simulink model "friction_compensation_test"  (R2022b)
settings: Solver=VariableStepAuto  StartTime=0.0  StopTime=10.0  RelTol=1e-3
values from neighbouring files (symbols this model uses):
  error_min = 0.04    [matlab.mat]
  pwm_k = 0.02    [matlab.mat]
  pwm_min = 0.27    [matlab.mat]
settings Model: Creator=sjohnson  LastModifiedBy=sjohnson

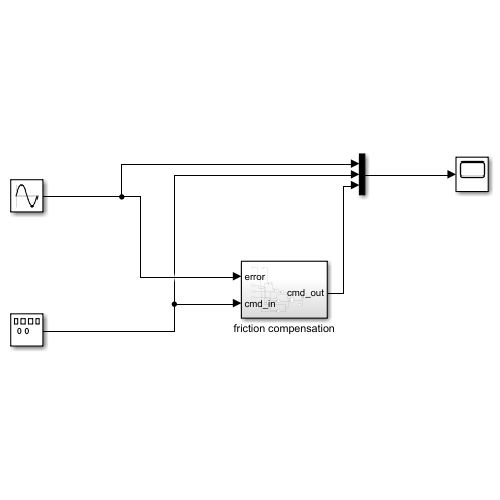
[thumbnail: Simulink's stored preview of the top-level diagram]
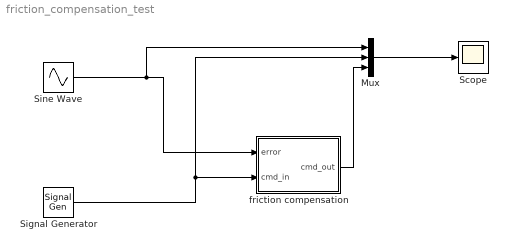
== system friction_compensation_test ==
  Mux : Mux  Inputs=3
  Scope : Scope
  Signal Generator : SignalGenerator  WaveForm=sawtooth  Units=rad/sec
  Sine Wave : Sin  SampleTime=0
  friction compensation : Subsystem
  wires:
  Sine Wave/1 -> Mux/1, friction compensation/1(error)
  Signal Generator/1 -> Mux/2, friction compensation/2(cmd_in)
  friction compensation/1(cmd_out) -> Mux/3
  Mux/1 -> Scope/1

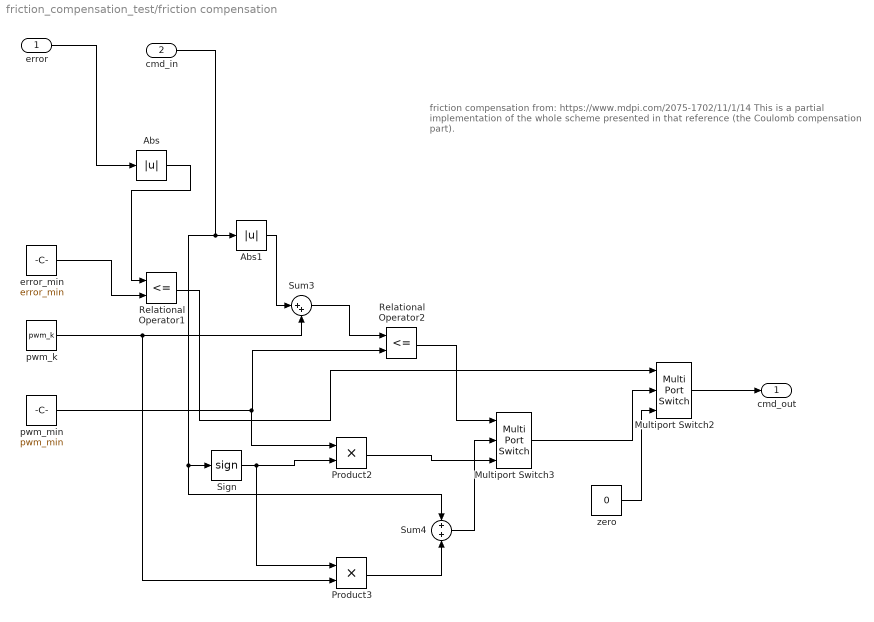
== system friction_compensation_test/friction compensation ==
  note: friction compensation from:
      | https://www.mdpi.com/2075-1702/11/1/14
      | This is a partial implementation of the whole scheme presented in that reference (the Coulomb compensation part).
  error : Inport
  cmd_in : Inport  Port=2
  Abs : Abs  SaturateOnIntegerOverflow=off
  Abs1 : Abs  SaturateOnIntegerOverflow=off
  Multiport Switch2 : MultiPortSwitch  DataPortOrder=Zero-based contiguous  Inputs=2  zeroidx=on  SaturateOnIntegerOverflow=off  InputSameDT=off
  Multiport Switch3 : MultiPortSwitch  DataPortOrder=Zero-based contiguous  Inputs=2  zeroidx=on  SaturateOnIntegerOverflow=off  InputSameDT=off
  Product2 : Product
  Product3 : Product
  Relational Operator1 : RelationalOperator  Operator=<=  OutDataTypeStr=boolean  RndMeth=Simplest  InputSameDT=off
  Relational Operator2 : RelationalOperator  Operator=<=  OutDataTypeStr=boolean  RndMeth=Simplest  InputSameDT=off
  Sign : Signum
  Sum3 : Sum  Inputs=|++
  Sum4 : Sum
  error_min : Constant  Value=error_min
  pwm_k : Constant  Value=pwm_k
  pwm_min : Constant  Value=pwm_min
  zero : Constant  Value=0
  cmd_out : Outport
  wires:
  cmd_in/1 -> Sum4/1, Sign/1, Abs1/1
  Relational Operator1/1 -> Multiport Switch2/1
  zero/1 -> Multiport Switch2/3
  Sum3/1 -> Relational Operator2/1
  Product2/1 -> Multiport Switch3/3
  Sign/1 -> Product3/1, Product2/2
  Product3/1 -> Sum4/2
  Relational Operator2/1 -> Multiport Switch3/1
  Multiport Switch2/1 -> cmd_out/1
  error/1 -> Abs/1
  pwm_min/1 -> Product2/1, Relational Operator2/2
  error_min/1 -> Relational Operator1/2
  pwm_k/1 -> Product3/2, Sum3/2
  Abs/1 -> Relational Operator1/1
  Abs1/1 -> Sum3/1
  Multiport Switch3/1 -> Multiport Switch2/2
  Sum4/1 -> Multiport Switch3/2
